simulink library "Diesel_Genset_lib"  (R2013a)
settings: Solver=ode45  StartTime=0.0  StopTime=10.0  RelTol=1e-3
undefined symbols (not defined in the file or in its folder): DiscIntNeverNeededParam, fdesignblkfcn, gcbh, ph, Ts
libraries: simulink x19, rtio_opalrt_common x19, powerlib x18, discretizing x4, rteventslib x4, simulink_extras x3, powerlib_extras x1, NG_Genset_lib x1
(part 1 of 3)
settings Model: Creator=ed12083  LastModifiedBy=ed12083

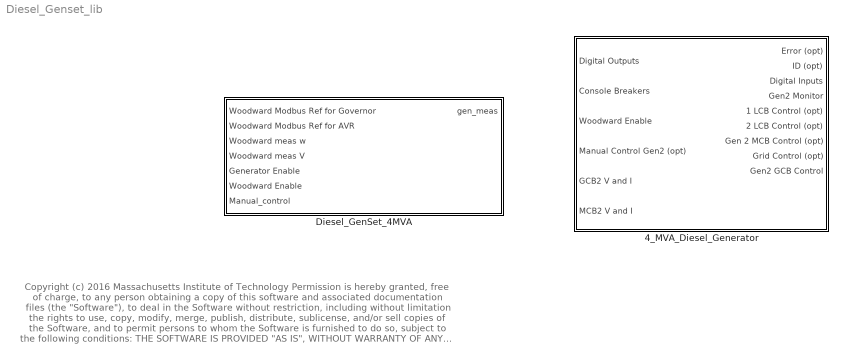
== system Diesel_Genset_lib ==
  note: Copyright (c) 2016 Massachusetts Institute of Technology
      | Permission is hereby granted, free of charge, to any person obtaining a copy of this software and associated documentation files (the "Software"), to deal
      | in the Software without restriction, including without limitation the rights to use, copy, modify, merge, publish, distribute, sublicense, and/or sell copies of the
      | Software, and to permit persons to whom the Software is furnished to do so, subject to the following conditions:
      |
      | THE SOFTWARE IS PROVIDED "AS IS", WITHOUT WARRANTY OF ANY KIND, EXPRESS OR IMPLIED, INCLUDING BUT NOT LIMITED TO THE
      | WARRANTIES OF MERCHANTABILITY, FITNESS FOR A PARTICULAR PURPOSE AND NONINFRINGEMENT. IN NO EVENT SHALL THE AUTHORS
      | OR COPYRIGHT HOLDERS BE LIABLE FOR ANY CLAIM, DAMAGES OR OTHER LIABILITY, WHETHER IN AN ACTION OF CONTRACT, TORT OR
      | OTHERWISE, ARISING FROM, OUT OF OR IN CONNECTION WITH THE SOFTWARE OR THE USE OR OTHER DEALINGS IN THE SOFTWARE.
  4_MVA_Diesel_Generator : Subsystem
  Diesel_GenSet_4MVA : Subsystem  mask(Gen-Set with simulated control modes){control_mode=1}
      mask prompts: control_mode "Control Mode [0 => Sim. 1 => Wood.]"
      mask help:
      | This Gen-Set block allows the user to indicate the control mode of the generator. The available control modes are: (1) PQ, (2) PV, and (3) VF.
      | The input values to the block will be applied according to the selected control mode.
      | For example, if PQ mode is selected, the controller will only work based on P_ref and Q_ref ignoring values of other inputs to the block.

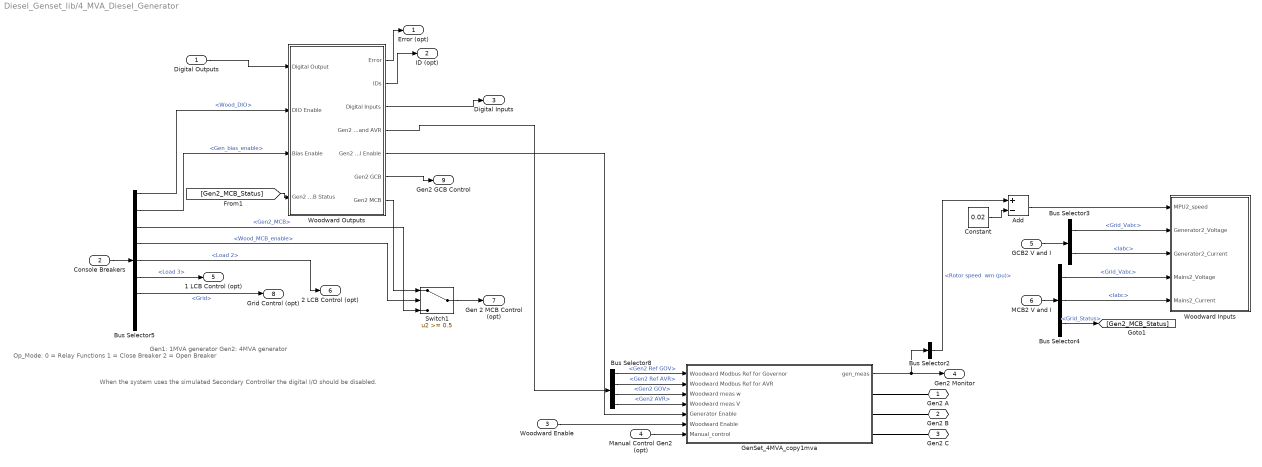
== system Diesel_Genset_lib/4_MVA_Diesel_Generator ==
  note: When the system uses the simulated
      | Secondary Controller the digital I/O
      | should be disabled.
  note: Gen1: 1MVA generator
      | Gen2: 4MVA generator
  note: Op_Mode:
      | 0 = Relay Functions
      | 1 = Close Breaker
      | 2 = Open Breaker
  Digital Outputs : Inport
  Console Breakers : Inport  Port=2
  Woodward Enable : Inport  Port=3
  Manual Control Gen2 (opt) : Inport  Port=4
  GCB2 V and I : Inport  Port=5
  MCB2 V and I : Inport  Port=6
  Add : Sum  Inputs=+-
  Bus Selector2 : BusSelector  OutputSignals="w.w.Rotor speed  wm (pu)"
  Bus Selector3 : BusSelector  OutputSignals=sel_787.Grid_Vabc,sel_787.Iabc
  Bus Selector4 : BusSelector  OutputSignals=sel_787.Grid_Vabc,sel_787.Iabc,Grid_Status
  Bus Selector5 : BusSelector  OutputSignals=Wood_DIO,Gen_bias_enable,Gen2_MCB,Wood_MCB_enable,Load 2,Load 3,Grid,Gen2_enable,Load 1
  Bus Selector8 : BusSelector  OutputSignals=Gen2 Ref GOV,Gen2 Ref AVR,Gen2 GOV,Gen2 AVR
  Constant : Constant  Value=0.02
  GenSet_4MVA_copy1mva : Subsystem  mask(Gen-Set with simulated control modes){control_mode=1}
      mask prompts: control_mode "Control Mode [0 => Sim. 1 => Wood.]"
      mask help:
      | This Gen-Set block allows the user to indicate the control mode of the generator. The available control modes are: (1) PQ, (2) PV, and (3) VF.
      | The input values to the block will be applied according to the selected control mode.
      | For example, if PQ mode is selected, the controller will only work based on P_ref and Q_ref ignoring values of other inputs to the block.
  Switch1 : Switch  Threshold=0.5
  Woodward Inputs : Subsystem
  Woodward Outputs : Subsystem
  Gen2 A : PMIOPort  Port=1  Side=Right
  Gen2 B : PMIOPort  Port=2  Side=Right
  Gen2 C : PMIOPort  Port=3  Side=Right
  Error (opt) : Outport
  ID (opt) : Outport  Port=2
  Digital Inputs : Outport  Port=3
  Gen2 Monitor : Outport  Port=4
  1 LCB Control (opt) : Outport  Port=5
  2 LCB Control (opt) : Outport  Port=6
  Gen 2 MCB Control (opt) : Outport  Port=7
  Grid Control (opt) : Outport  Port=8
  Gen2 GCB Control : Outport  Port=9
  wires:
  Bus Selector2/1 -> Add/1  "<Rotor speed  wm (pu)>"
  Bus Selector5/7 -> Grid Control (opt)/1  "<Grid>"
  Bus Selector5/3 -> Switch1/3  "<Gen2_MCB>"
  Bus Selector5/5 -> 2 LCB Control (opt)/1  "<Load 2>"
  Woodward Outputs/7(Gen2 MCB) -> Switch1/1
  Switch1/1 -> Gen 2 MCB Control (opt)/1
  [Gen2_MCB_Status] -> Woodward Outputs/4(Gen2 MCB Status)
  Bus Selector4/3 -> [Gen2_MCB_Status]  "<Grid_Status>"
  Constant/1 -> Add/2
  Add/1 -> Woodward Inputs/1(MPU2_speed)
  Woodward Outputs/6(Gen2 GCB) -> Gen2 GCB Control/1
  Woodward Outputs/5(Gen2 Fuel Enable) -> GenSet_4MVA_copy1mva/5(Generator Enable)
  Manual Control Gen2 (opt)/1 -> GenSet_4MVA_copy1mva/7(Manual_control)
  Bus Selector8/4 -> GenSet_4MVA_copy1mva/4(Woodward meas V)  "<Gen2 AVR>"
  Bus Selector8/3 -> GenSet_4MVA_copy1mva/3(Woodward meas w)  "<Gen2 GOV>"
  Bus Selector8/2 -> GenSet_4MVA_copy1mva/2(Woodward Modbus Ref for AVR)  "<Gen2 Ref AVR>"
  Bus Selector8/1 -> GenSet_4MVA_copy1mva/1(Woodward Modbus Ref for Governor)  "<Gen2 Ref GOV>"
  Woodward Outputs/4(Gen2 Gov and AVR) -> Bus Selector8/1
  Bus Selector4/2 -> Woodward Inputs/5(Mains2_Current)  "<Iabc>"
  Bus Selector4/1 -> Woodward Inputs/4(Mains2_Voltage)  "<Grid_Vabc>"
  Bus Selector3/2 -> Woodward Inputs/3(Generator2_Current)  "<Iabc>"
  Bus Selector3/1 -> Woodward Inputs/2(Generator2_Voltage)  "<Grid_Vabc>"
  GenSet_4MVA_copy1mva/1(gen_meas) -> Gen2 Monitor/1, Bus Selector2/1
  MCB2 V and I/1 -> Bus Selector4/1
  GCB2 V and I/1 -> Bus Selector3/1
  Bus Selector5/6 -> 1 LCB Control (opt)/1  "<Load 3>"
  Console Breakers/1 -> Bus Selector5/1
  Digital Outputs/1 -> Woodward Outputs/1(Digital Output)
  Bus Selector5/4 -> Switch1/2  "<Wood_MCB_enable>"
  Woodward Enable/1 -> GenSet_4MVA_copy1mva/6(Woodward Enable)
  Woodward Outputs/3(Digital Inputs) -> Digital Inputs/1
  Woodward Outputs/2(IDs) -> ID (opt)/1
  Woodward Outputs/1(Error) -> Error (opt)/1
  Bus Selector5/2 -> Woodward Outputs/3(Bias Enable)  "<Gen_bias_enable>"
  Bus Selector5/1 -> Woodward Outputs/2(DIO Enable)  "<Wood_DIO>"
  connections:
  Gen2 C/RConn1 -- GenSet_4MVA_copy1mva/RConn3
  GenSet_4MVA_copy1mva/RConn2 -- Gen2 B/RConn1
  Gen2 A/RConn1 -- GenSet_4MVA_copy1mva/RConn1

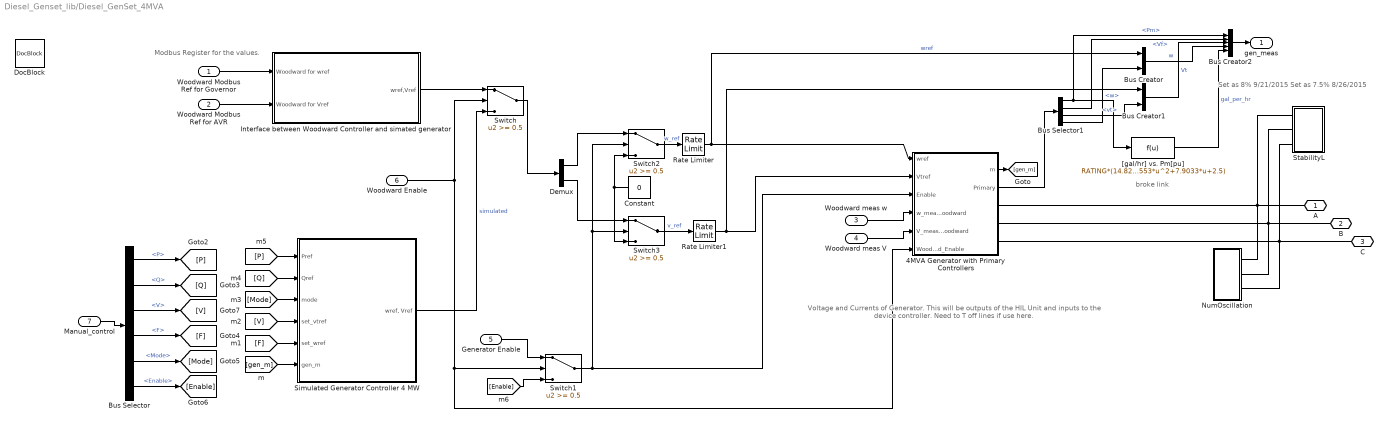
== system Diesel_Genset_lib/Diesel_GenSet_4MVA ==
  note: Modbus Register for the values.
  note: Voltage and Currents of Generator.
      | This will be outputs of the HIL Unit
      | and inputs to the device controller.
      | Need to T off lines if use here.
  note: Set as 8% 9/21/2015
      | Set as 7.5% 8/26/2015
  note: broke link
  Woodward Modbus Ref for Governor : Inport
  Woodward Modbus Ref for AVR : Inport  Port=2
  Woodward meas w : Inport  Port=3
  Woodward meas V : Inport  Port=4
  Generator Enable : Inport  Port=5
  Woodward Enable : Inport  Port=6
  Manual_control : Inport  Port=7
  4MVA Generator with Primary Controllers : Subsystem
  Bus Creator : BusCreator  Inputs=2
  Bus Creator1 : BusCreator  Inputs=2
  Bus Creator2 : BusCreator  Inputs=5
  Bus Selector : BusSelector  OutputSignals=P,Q,V,F,Mode,Enable
  Bus Selector1 : BusSelector  OutputSignals=Pm,Vf,vt,w
  Constant : Constant  Value=0
  Demux : Demux  Outputs=2
  DocBlock : simulink/Model-Wide Utilities/DocBlock  DocumentType=Text
      content=|
      | Author: Mirjana Marden, May 2015
      |
      | This is the model of 60kW generator with AVR and Governor.
      | There are two modes for controller implementation:
      |     1. Hardware implemented Woodward controller
      |     2. Simulated Generator Controller
      |
      | 1. Hardware implemented Woodward controller's output signals are DC voltages for both bias signals.
      |    The voltage range is -10 to 10V.
      |    The commanded reference values for generator frequency and voltage are wref and Vref.
      |    Interface between Woodward controller and simulation is a block that scales the bias signals.
      | 2. Simulated generator controller has three modes PQ, Vf and PV
  Interface between Woodward Controller and simated generator : Subsystem
  NumOscillation : Subsystem
  Rate Limiter : RateLimiter  RisingSlewLimit=0.5  FallingSlewLimit=-0.5  SampleTimeMode=inherited
  Rate Limiter1 : RateLimiter  RisingSlewLimit=0.5  FallingSlewLimit=-0.5  SampleTimeMode=inherited
  Simulated Generator Controller 4 MW : Subsystem
  StabilityL : Subsystem  mask{v=13800, kVA=320, pf=1}
  Switch{,1..3} (4 alike) : Switch  Threshold=0.5
  "[gal/hr] vs. Pm[pu]" : Fcn  Expr=RATING*(14.827*u^4-27.253*u^3+15.553*u^2+7.9033*u+2.5)  mask{RATING=4}
      mask prompts: RATING "Rating [MW]"
      mask help: This block computes the gal/hr vs Pm[pu] of a generator of a given rating [MW].
  A : PMIOPort  Port=1  Side=Right
  B : PMIOPort  Port=2  Side=Right
  C : PMIOPort  Port=3  Side=Right
  gen_meas : Outport
  wires:
  [F] -> Simulated Generator Controller 4 MW/5(set_wref)
  [V] -> Simulated Generator Controller 4 MW/4(set_vtref)
  [Mode] -> Simulated Generator Controller 4 MW/3(mode)
  [Q] -> Simulated Generator Controller 4 MW/2(Qref)
  [P] -> Simulated Generator Controller 4 MW/1(Pref)
  [gen_m] -> Simulated Generator Controller 4 MW/6(gen_m)
  Bus Selector/5 -> [Mode]  "<Mode>"
  Bus Selector/4 -> [F]  "<F>"
  Bus Selector/3 -> [V]  "<V>"
  Bus Selector/2 -> [Q]  "<Q>"
  Bus Selector/1 -> [P]  "<P>"
  Manual_control/1 -> Bus Selector/1
  Simulated Generator Controller 4 MW/1("wref, Vref") -> Switch/3  "simulated"
  4MVA Generator with Primary Controllers/1(m) -> [gen_m]
  Interface between Woodward Controller and simated generator/1(wref,Vref) -> Switch/1
  Switch/1 -> Demux/1
  Woodward Modbus Ref for Governor/1 -> Interface between Woodward Controller and simated generator/1(Woodward for wref)
  Woodward Modbus Ref for AVR/1 -> Interface between Woodward Controller and simated generator/2(Woodward for Vref)
  Woodward meas w/1 -> 4MVA Generator with Primary Controllers/4(w_meas_Woodward)
  Woodward meas V/1 -> 4MVA Generator with Primary Controllers/5(V_meas_Woodward)
  Bus Selector/6 -> [Enable]  "<Enable>"
  4MVA Generator with Primary Controllers/2(Primary) -> Bus Selector1/1
  Generator Enable/1 -> Switch1/1
  [Enable] -> Switch1/3
  Switch1/1 -> 4MVA Generator with Primary Controllers/3(Enable), Switch2/2, Switch3/2
  Switch2/1 -> Rate Limiter/1  "w_ref"
  Demux/1 -> Switch2/1
  Demux/2 -> Switch3/1
  Constant/1 -> Switch3/3, Switch2/3
  Switch3/1 -> Rate Limiter1/1  "v_ref"
  Bus Selector1/3 -> Bus Creator1/2  "<vt>"
  Bus Selector1/4 -> Bus Creator/2  "<w>"
  Bus Selector1/2 -> Bus Creator2/2  "<Vf>"
  Bus Selector1/1 -> Bus Creator2/1, "[gal/hr] vs. Pm[pu]"/1  "<Pm>"
  Bus Creator1/1 -> Bus Creator2/3  "Vt"
  Bus Creator/1 -> Bus Creator2/4  "w"
  Bus Creator2/1 -> gen_meas/1
  Rate Limiter/1 -> 4MVA Generator with Primary Controllers/1(wref), Bus Creator/1  "wref"
  Rate Limiter1/1 -> 4MVA Generator with Primary Controllers/2(Vtref), Bus Creator1/1
  Woodward Enable/1 -> Switch/2, Switch1/2, 4MVA Generator with Primary Controllers/6(Woodward_Enable)
  "[gal/hr] vs. Pm[pu]"/1 -> Bus Creator2/5  "gal_per_hr"
  connections:
  StabilityL/LConn1 -- A/RConn1 -- 4MVA Generator with Primary Controllers/RConn1 -- NumOscillation/LConn1
  StabilityL/LConn2 -- 4MVA Generator with Primary Controllers/RConn2 -- B/RConn1 -- NumOscillation/LConn2
  StabilityL/LConn3 -- C/RConn1 -- 4MVA Generator with Primary Controllers/RConn3 -- NumOscillation/LConn3

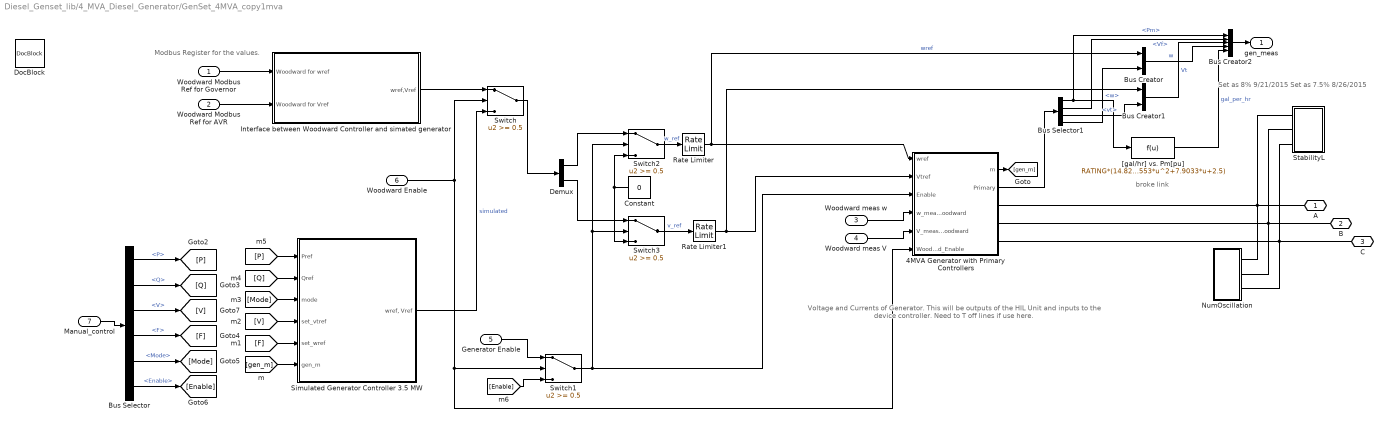
== system Diesel_Genset_lib/4_MVA_Diesel_Generator/GenSet_4MVA_copy1mva ==
  note: Modbus Register for the values.
  note: Voltage and Currents of Generator.
      | This will be outputs of the HIL Unit
      | and inputs to the device controller.
      | Need to T off lines if use here.
  note: Set as 8% 9/21/2015
      | Set as 7.5% 8/26/2015
  note: broke link
  Woodward Modbus Ref for Governor : Inport
  Woodward Modbus Ref for AVR : Inport  Port=2
  Woodward meas w : Inport  Port=3
  Woodward meas V : Inport  Port=4
  Generator Enable : Inport  Port=5
  Woodward Enable : Inport  Port=6
  Manual_control : Inport  Port=7
  4MVA Generator with Primary Controllers : Subsystem
  Bus Creator : BusCreator  Inputs=2
  Bus Creator1 : BusCreator  Inputs=2
  Bus Creator2 : BusCreator  Inputs=5
  Bus Selector : BusSelector  OutputSignals=P,Q,V,F,Mode,Enable
  Bus Selector1 : BusSelector  OutputSignals=Pm,Vf,vt,w
  Constant : Constant  Value=0
  Demux : Demux  Outputs=2
  DocBlock : simulink/Model-Wide Utilities/DocBlock  DocumentType=Text
      content=|
      | Author: Mirjana Marden, May 2015
      |
      | This is the model of 60kW generator with AVR and Governor.
      | There are two modes for controller implementation:
      |     1. Hardware implemented Woodward controller
      |     2. Simulated Generator Controller
      |
      | 1. Hardware implemented Woodward controller's output signals are DC voltages for both bias signals.
      |    The voltage range is -10 to 10V.
      |    The commanded reference values for generator frequency and voltage are wref and Vref.
      |    Interface between Woodward controller and simulation is a block that scales the bias signals.
      | 2. Simulated generator controller has three modes PQ, Vf and PV
  Interface between Woodward Controller and simated generator : Subsystem
  NumOscillation : Subsystem
  Rate Limiter : RateLimiter  RisingSlewLimit=0.5  FallingSlewLimit=-0.5  SampleTimeMode=inherited
  Rate Limiter1 : RateLimiter  RisingSlewLimit=0.5  FallingSlewLimit=-0.5  SampleTimeMode=inherited
  Simulated Generator Controller 3.5 MW : Subsystem
  StabilityL : Subsystem  mask{v=13800, kVA=320, pf=1}
  Switch{,1..3} (4 alike) : Switch  Threshold=0.5
  "[gal/hr] vs. Pm[pu]" : Fcn  Expr=RATING*(14.827*u^4-27.253*u^3+15.553*u^2+7.9033*u+2.5)  mask{RATING=4}
      mask prompts: RATING "Rating [MW]"
      mask help: This block computes the gal/hr vs Pm[pu] of a generator of a given rating [MW].
  A : PMIOPort  Port=1  Side=Right
  B : PMIOPort  Port=2  Side=Right
  C : PMIOPort  Port=3  Side=Right
  gen_meas : Outport
  wires:
  [F] -> Simulated Generator Controller 3.5 MW/5(set_wref)
  [V] -> Simulated Generator Controller 3.5 MW/4(set_vtref)
  [Mode] -> Simulated Generator Controller 3.5 MW/3(mode)
  [Q] -> Simulated Generator Controller 3.5 MW/2(Qref)
  [P] -> Simulated Generator Controller 3.5 MW/1(Pref)
  [gen_m] -> Simulated Generator Controller 3.5 MW/6(gen_m)
  Bus Selector/5 -> [Mode]  "<Mode>"
  Bus Selector/4 -> [F]  "<F>"
  Bus Selector/3 -> [V]  "<V>"
  Bus Selector/2 -> [Q]  "<Q>"
  Bus Selector/1 -> [P]  "<P>"
  Manual_control/1 -> Bus Selector/1
  Simulated Generator Controller 3.5 MW/1("wref, Vref") -> Switch/3  "simulated"
  4MVA Generator with Primary Controllers/1(m) -> [gen_m]
  Interface between Woodward Controller and simated generator/1(wref,Vref) -> Switch/1
  Switch/1 -> Demux/1
  Woodward Modbus Ref for Governor/1 -> Interface between Woodward Controller and simated generator/1(Woodward for wref)
  Woodward Modbus Ref for AVR/1 -> Interface between Woodward Controller and simated generator/2(Woodward for Vref)
  Woodward meas w/1 -> 4MVA Generator with Primary Controllers/4(w_meas_Woodward)
  Woodward meas V/1 -> 4MVA Generator with Primary Controllers/5(V_meas_Woodward)
  Bus Selector/6 -> [Enable]  "<Enable>"
  4MVA Generator with Primary Controllers/2(Primary) -> Bus Selector1/1
  Generator Enable/1 -> Switch1/1
  [Enable] -> Switch1/3
  Switch1/1 -> 4MVA Generator with Primary Controllers/3(Enable), Switch2/2, Switch3/2
  Switch2/1 -> Rate Limiter/1  "w_ref"
  Demux/1 -> Switch2/1
  Demux/2 -> Switch3/1
  Constant/1 -> Switch3/3, Switch2/3
  Switch3/1 -> Rate Limiter1/1  "v_ref"
  Bus Selector1/3 -> Bus Creator1/2  "<vt>"
  Bus Selector1/4 -> Bus Creator/2  "<w>"
  Bus Selector1/2 -> Bus Creator2/2  "<Vf>"
  Bus Selector1/1 -> Bus Creator2/1, "[gal/hr] vs. Pm[pu]"/1  "<Pm>"
  Bus Creator1/1 -> Bus Creator2/3  "Vt"
  Bus Creator/1 -> Bus Creator2/4  "w"
  Bus Creator2/1 -> gen_meas/1
  Rate Limiter/1 -> 4MVA Generator with Primary Controllers/1(wref), Bus Creator/1  "wref"
  Rate Limiter1/1 -> 4MVA Generator with Primary Controllers/2(Vtref), Bus Creator1/1
  Woodward Enable/1 -> Switch/2, Switch1/2, 4MVA Generator with Primary Controllers/6(Woodward_Enable)
  "[gal/hr] vs. Pm[pu]"/1 -> Bus Creator2/5  "gal_per_hr"
  connections:
  StabilityL/LConn1 -- A/RConn1 -- 4MVA Generator with Primary Controllers/RConn1 -- NumOscillation/LConn1
  StabilityL/LConn2 -- 4MVA Generator with Primary Controllers/RConn2 -- B/RConn1 -- NumOscillation/LConn2
  StabilityL/LConn3 -- C/RConn1 -- 4MVA Generator with Primary Controllers/RConn3 -- NumOscillation/LConn3

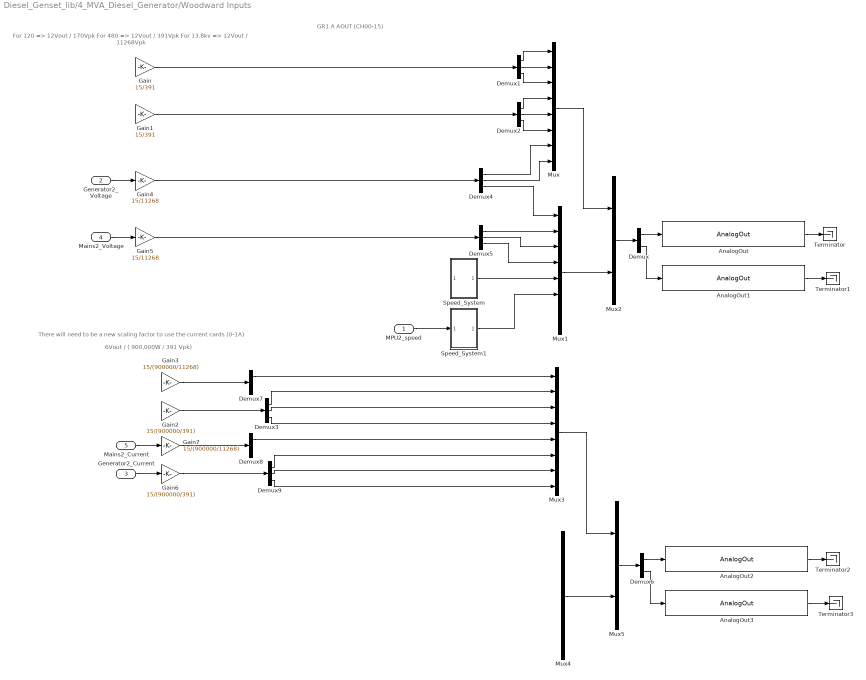
== system Diesel_Genset_lib/4_MVA_Diesel_Generator/Woodward Inputs ==
  note: There will need to be a
      | new scaling factor to use
      | the current cards (0-1A)
  note: GR1 A AOUT (CH00-15)
  note: For 120 => 12Vout / 170Vpk
      | For 480 => 12Vout / 391Vpk
      | For 13.8kv => 12Vout / 11268Vpk
  note: 6Vout / ( 900,000W / 391 Vpk)
  MPU2_speed : Inport
  Generator2_Voltage : Inport  Port=2
  Generator2_Current : Inport  Port=3
  Mains2_Voltage : Inport  Port=4
  Mains2_Current : Inport  Port=5
  AnalogOut : rtio_opalrt_common/AnalogOut  CtrlName='OpCtrl'  portNb=1  FcnNos=Slot 1 Module A Subsection 1  size=16  maxcount=8  count=8  numchan=8  israngeinput=off  voltagerange=[-16 ... 16]  slot=0  side=0  mismatch=0  slotside=Slot_1_Module_A
      settings: AttributesFormatString=%<CtrlName>
  AnalogOut1 : rtio_opalrt_common/AnalogOut  CtrlName='OpCtrl'  portNb=2  FcnNos=Slot 1 Module A Subsection 2  size=16  maxcount=8  count=8  numchan=8  israngeinput=off  voltagerange=[-16 ... 16]  slot=0  side=0  mismatch=0  slotside=Slot_1_Module_A
      settings: AttributesFormatString=%<CtrlName>
  AnalogOut2 : rtio_opalrt_common/AnalogOut  CtrlName='OpCtrl'  portNb=3  FcnNos=Slot 2 Module A Subsection 1  size=16  maxcount=8  count=8  numchan=8  israngeinput=off  voltagerange=[-16 ... 16]  slot=1  side=0  mismatch=0  slotside=Slot_2_Module_A
      settings: AttributesFormatString=%<CtrlName>
  AnalogOut3 : rtio_opalrt_common/AnalogOut  CtrlName='OpCtrl'  portNb=4  FcnNos=Slot 2 Module A Subsection 2  size=16  maxcount=8  count=8  numchan=8  israngeinput=off  voltagerange=[-16 ... 16]  slot=1  side=0  mismatch=0  slotside=Slot_2_Module_A
      settings: AttributesFormatString=%<CtrlName>
  Demux : Demux  Outputs=2
  Demux{1..5,7..9} (8 alike) : Demux  Outputs=3
  Demux6 : Demux  Outputs=2
  Gain : Gain  Gain=15/391
  Gain1 : Gain  Gain=15/391
  Gain2 : Gain  Gain=15/(900000/391)
  Gain3 : Gain  Gain=15/(900000/11268)
  Gain4 : Gain  Gain=15/11268
  Gain5 : Gain  Gain=15/11268
  Gain6 : Gain  Gain=15/(900000/391)
  Gain7 : Gain  Gain=15/(900000/11268)
  Mux{,1,3..4} (4 alike) : Mux  Inputs=8
  Mux2 : Mux  Inputs=2
  Mux5 : Mux  Inputs=2
  Speed_System : Subsystem
  Speed_System1 : Subsystem
  Terminator{,1..3} (4 alike) : Terminator
  wires:
  Demux9/3 -> Mux3/8
  Demux9/2 -> Mux3/7
  Demux9/1 -> Mux3/6
  Gain6/1 -> Demux9/1
  Demux8/1 -> Mux3/5
  Gain7/1 -> Demux8/1
  Mains2_Current/1 -> Gain7/1
  Generator2_Current/1 -> Gain6/1
  Speed_System1/1(Out1) -> Mux1/6
  MPU2_speed/1 -> Speed_System1/1(In1)
  Generator2_Voltage/1 -> Gain4/1
  Mains2_Voltage/1 -> Gain5/1
  Gain4/1 -> Demux4/1
  Gain5/1 -> Demux5/1
  Demux7/1 -> Mux3/1
  Gain3/1 -> Demux7/1
  ? -> Gain3/1
  Demux3/3 -> Mux3/4
  Demux3/2 -> Mux3/3
  Demux3/1 -> Mux3/2
  Gain2/1 -> Demux3/1
  AnalogOut2/1 -> Terminator2/1
  AnalogOut3/1 -> Terminator3/1
  Demux6/1 -> AnalogOut2/1
  Demux6/2 -> AnalogOut3/1
  Mux3/1 -> Mux5/1
  Mux4/1 -> Mux5/2
  Mux5/1 -> Demux6/1
  Demux5/3 -> Mux1/4
  Demux5/2 -> Mux1/3
  Demux5/1 -> Mux1/2
  Demux4/3 -> Mux1/1
  Demux4/2 -> Mux/8
  Demux4/1 -> Mux/7
  Speed_System/1(Out1) -> Mux1/5
  Demux2/3 -> Mux/6
  Demux2/2 -> Mux/5
  Demux2/1 -> Mux/4
  Demux1/3 -> Mux/3
  Demux1/2 -> Mux/2
  Demux1/1 -> Mux/1
  AnalogOut/1 -> Terminator/1
  AnalogOut1/1 -> Terminator1/1
  Demux/1 -> AnalogOut/1
  Demux/2 -> AnalogOut1/1
  ? -> Gain/1
  Mux/1 -> Mux2/1
  Mux1/1 -> Mux2/2
  Mux2/1 -> Demux/1
  ? -> Gain1/1
  Gain/1 -> Demux1/1
  Gain1/1 -> Demux2/1
  ? -> Gain2/1
  ? -> Speed_System/1(In1)

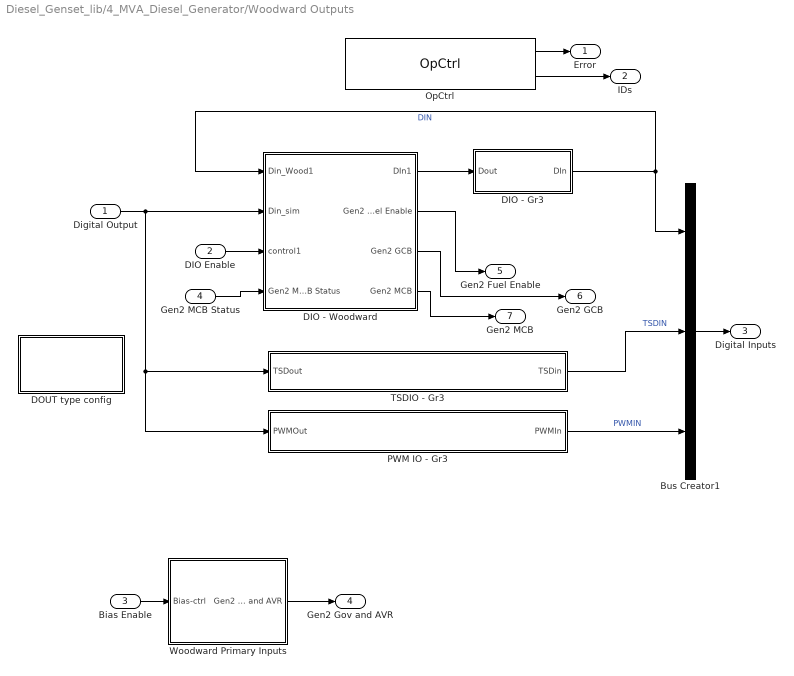
== system Diesel_Genset_lib/4_MVA_Diesel_Generator/Woodward Outputs ==
  Digital Output : Inport
  DIO Enable : Inport  Port=2
  Bias Enable : Inport  Port=3
  Gen2 MCB Status : Inport  Port=4
  Bus Creator1 : BusCreator  Inputs=3
  DIO - Gr3 : Subsystem
  DIO - Woodward : Subsystem
  DOUT type config : Subsystem
  OpCtrl : rtio_opalrt_common/OpCtrl  CtrlName='OpCtrl'  boardid=0  BitstreamFilename=VC707_2-EX-0001-2_2_6_61-32AIO16DIO16DIOSel-01-01.bin  numconfig=-1  mode=Master  externalClock=off  decimRtsi=0  calibIO=off  SampleTime=0  loadinport=-1  BoardType=VC707  SecondaryPresent=off  sync_type=Audio
  PWM IO - Gr3 : Subsystem
  TSDIO - Gr3 : Subsystem
  Woodward Primary Inputs : Subsystem
  Error : Outport
  IDs : Outport  Port=2
  Digital Inputs : Outport  Port=3
  Gen2 Gov and AVR : Outport  Port=4
  Gen2 Fuel Enable : Outport  Port=5
  Gen2 GCB : Outport  Port=6
  Gen2 MCB : Outport  Port=7
  wires:
  Gen2 MCB Status/1 -> DIO - Woodward/4(Gen2 MCB Status)
  DIO - Woodward/4(Gen2 MCB) -> Gen2 MCB/1
  DIO - Woodward/2(Gen2 Fuel Enable) -> Gen2 Fuel Enable/1
  DIO - Woodward/3(Gen2 GCB) -> Gen2 GCB/1
  Digital Output/1 -> TSDIO - Gr3/1(TSDout), PWM IO - Gr3/1(PWMOut), DIO - Woodward/2(Din_sim)
  Bias Enable/1 -> Woodward Primary Inputs/1(Bias-ctrl)
  Woodward Primary Inputs/1(Gen2 Gov and AVR) -> Gen2 Gov and AVR/1
  DIO Enable/1 -> DIO - Woodward/3(control1)
  Bus Creator1/1 -> Digital Inputs/1
  DIO - Gr3/1(DIn) -> DIO - Woodward/1(Din_Wood1), Bus Creator1/1  "DIN"
  TSDIO - Gr3/1(TSDin) -> Bus Creator1/2  "TSDIN"
  PWM IO - Gr3/1(PWMIn) -> Bus Creator1/3  "PWMIN"
  DIO - Woodward/1(DIn1) -> DIO - Gr3/1(Dout)
  OpCtrl/2 -> IDs/1
  OpCtrl/1 -> Error/1

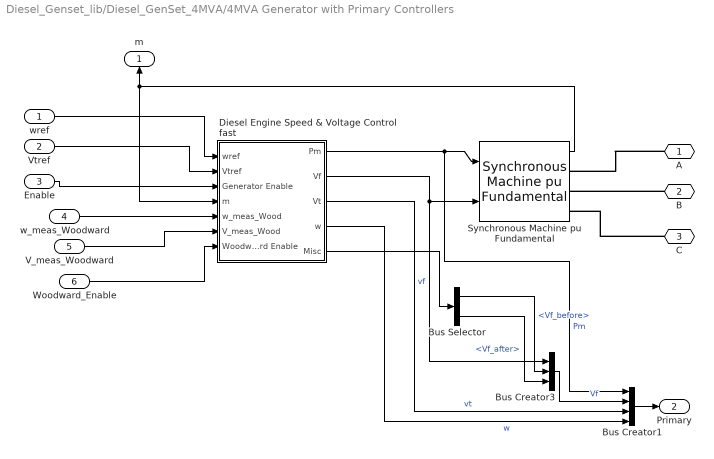
== system Diesel_Genset_lib/Diesel_GenSet_4MVA/4MVA Generator with Primary Controllers ==
  wref : Inport
  Vtref : Inport  Port=2
  Enable : Inport  Port=3
  w_meas_Woodward : Inport  Port=4
  V_meas_Woodward : Inport  Port=5
  Woodward_Enable : Inport  Port=6
  Bus Creator1 : BusCreator
  Bus Creator3 : BusCreator  Inputs=3
  Bus Selector : BusSelector  OutputSignals=Vf_before,Vf_after
  Diesel Engine Speed & Voltage Control fast : Subsystem
  Synchronous Machine pu Fundamental : powerlib/Machines/Synchronous Machine pu Fundamental  PresetModel=No  MechanicalLoad=Mechanical power Pm  ShowDetailedParameters=on  RotorType=Salient-pole  NominalParameters=[4e+006 13800 60]  Stator=[0.008979 0.05 2.35 1.72]  Field=[0.00206 0.511]  Dampers2=[0.0652, 0.5134, 0.0287, 0.2553, 7.765e-3, 0.9167 ]  Dampers1=[0.2826 3.738 0.02545 0.2392]  Mechanical=[0.3468 0.009238 2]  PolePairs=2  InitialConditions="[ -99  0  0  0  0  0  0  0  0 ]"  SetSaturation=off  Saturation=[0.6404,0.7127,0.8441,0.9214,0.9956,1.082,1.19,1.316,1.457;0.7,0.7698,0.8872,0.9466,0.9969,1.046,1.1,1.151,1.201]  Units=per unit fundamental parameters  LoadFlowParameters=[1,0,0,0,0]  TsPowergui=0  TsBlock=-1  IterativeModel=Forward Euler  BusType=swing  Pref=0  Qref=0  Qmin=-inf  Qmax=inf  PLF=0  QLF=0
  A : PMIOPort  Port=1  Side=Right
  B : PMIOPort  Port=2  Side=Right
  C : PMIOPort  Port=3  Side=Right
  m : Outport
  Primary : Outport  Port=2
  wires:
  Vtref/1 -> Diesel Engine Speed & Voltage Control fast/2(Vtref)
  wref/1 -> Diesel Engine Speed & Voltage Control fast/1(wref)
  Diesel Engine Speed & Voltage Control fast/2(Vf) -> Synchronous Machine pu Fundamental/2, Bus Creator3/1  "vf"
  Diesel Engine Speed & Voltage Control fast/1(Pm) -> Synchronous Machine pu Fundamental/1, Bus Creator1/1  "Pm"
  Enable/1 -> Diesel Engine Speed & Voltage Control fast/3(Generator Enable)
  Synchronous Machine pu Fundamental/1 -> m/1, Diesel Engine Speed & Voltage Control fast/4(m)
  w_meas_Woodward/1 -> Diesel Engine Speed & Voltage Control fast/5(w_meas_Wood)
  V_meas_Woodward/1 -> Diesel Engine Speed & Voltage Control fast/6(V_meas_Wood)
  Diesel Engine Speed & Voltage Control fast/3(Vt) -> Bus Creator1/3  "vt"
  Diesel Engine Speed & Voltage Control fast/4(w) -> Bus Creator1/4  "w"
  Bus Creator1/1 -> Primary/1
  Diesel Engine Speed & Voltage Control fast/5(Misc) -> Bus Selector/1
  Bus Selector/1 -> Bus Creator3/2  "<Vf_before>"
  Bus Selector/2 -> Bus Creator3/3  "<Vf_after>"
  Bus Creator3/1 -> Bus Creator1/2  "Vf"
  Woodward_Enable/1 -> Diesel Engine Speed & Voltage Control fast/7(Woodward Enable)
  connections:
  C/RConn1 -- Synchronous Machine pu Fundamental/RConn3
  B/RConn1 -- Synchronous Machine pu Fundamental/RConn2
  A/RConn1 -- Synchronous Machine pu Fundamental/RConn1

== system Diesel_Genset_lib/Diesel_GenSet_4MVA/Interface between Woodward Controller and simated generator ==
  note: Note: This may need a different scaling because it is the reference signal.
      | Reference has to be between 0.95 and 1.05 pu in order to be in tolerance.
  Woodward for wref : Inport
  Woodward for Vref : Inport  Port=2
  Add2 : Sum
  Add3 : Sum
  Gain2 : Gain
  Gain3 : Gain
  Mux1 : Mux  Inputs=2
  Vref_set : Constant  Value=0
  wref_set : Constant  Value=0
  wref,Vref : Outport
  wires:
  Gain2/1 -> Add2/1  "bias"
  Add2/1 -> Mux1/1
  wref_set/1 -> Add2/2
  Gain3/1 -> Add3/1  "bias"
  Vref_set/1 -> Add3/2
  Add3/1 -> Mux1/2
  Woodward for wref/1 -> Gain2/1
  Mux1/1 -> wref,Vref/1  "hardware"
  Woodward for Vref/1 -> Gain3/1

== system Diesel_Genset_lib/Diesel_GenSet_4MVA/NumOscillation ==
  Ground2 : powerlib/Elements/Ground  LConnTagsString=a
  "RLC " : powerlib/Elements/Parallel RLC Branch  LConnTagsString=a  RConnTagsString=__new0  BranchType=R  Resistance=10e6  Inductance=inf  SetiL0=off  InitialCurrent=0  Capacitance=10e-6  Setx0=off  InitialVoltage=0  Measurements=None
  RLC1 : powerlib/Elements/Parallel RLC Branch  LConnTagsString=a  RConnTagsString=__new0  BranchType=R  Resistance=10e6  Inductance=inf  SetiL0=off  InitialCurrent=0  Capacitance=10e-6  Setx0=off  InitialVoltage=0  Measurements=None
  RLC2 : powerlib/Elements/Parallel RLC Branch  LConnTagsString=a  RConnTagsString=__new0  BranchType=R  Resistance=10e6  Inductance=inf  SetiL0=off  InitialCurrent=0  Capacitance=10e-6  Setx0=off  InitialVoltage=0  Measurements=None
  RLC3 : powerlib/Elements/Parallel RLC Branch  LConnTagsString=a  RConnTagsString=__new0  BranchType=R  Resistance=10e-3  Inductance=inf  SetiL0=off  InitialCurrent=0  Capacitance=0  Setx0=off  InitialVoltage=0  Measurements=None
  RLC4 : powerlib/Elements/Parallel RLC Branch  LConnTagsString=a  RConnTagsString=__new0  BranchType=R  Resistance=10e-3  Inductance=inf  SetiL0=off  InitialCurrent=0  Capacitance=0  Setx0=off  InitialVoltage=0  Measurements=None
  RLC5 : powerlib/Elements/Parallel RLC Branch  LConnTagsString=a  RConnTagsString=__new0  BranchType=R  Resistance=10e-3  Inductance=inf  SetiL0=off  InitialCurrent=0  Capacitance=0  Setx0=off  InitialVoltage=0  Measurements=None
  A : PMIOPort  Port=1  Side=Left
  B : PMIOPort  Port=2  Side=Left
  C : PMIOPort  Port=3  Side=Left
  connections:
  C/RConn1 -- RLC5/LConn1
  B/RConn1 -- RLC4/LConn1
  A/RConn1 -- RLC3/LConn1
  RLC3/RConn1 -- RLC2/LConn1
  RLC1/LConn1 -- RLC4/RConn1
  "RLC "/LConn1 -- RLC5/RConn1
  RLC2/RConn1 -- Ground2/LConn1 -- RLC1/RConn1 -- "RLC "/RConn1

== system Diesel_Genset_lib/Diesel_GenSet_4MVA/Simulated Generator Controller 4 MW ==
  Pref : Inport
  Qref : Inport  Port=2
  mode : Inport  Port=3
  set_vtref : Inport  Port=4
  set_wref : Inport  Port=5
  gen_m : Inport  Port=6
  Bus Selector1 : BusSelector  OutputSignals="Output active power   Peo (pu),Output reactive power  Qeo (pu)"
  Multiport Switch : MultiPortSwitch  DiagnosticForDefault=Warning
  Mux1 : Mux  Inputs=2
  Mux2 : Mux  Inputs=2
  Mux3 : Mux  Inputs=2
  PQ control : Subsystem
  PV control : Subsystem
  "wref, Vref" : Outport
  wires:
  Bus Selector1/1 -> PQ control/2(P (pu)), PV control/2(P (pu))  "<Output active power   Peo (pu)>"
  gen_m/1 -> Bus Selector1/1
  PQ control/1(w_ref (pu)) -> Mux1/1
  PQ control/2(V_ref (pu)) -> Mux1/2
  PV control/1(w_ref (pu)) -> Mux2/1
  set_vtref/1 -> Mux2/2, Mux3/2
  Mux1/1 -> Multiport Switch/2
  Mux2/1 -> Multiport Switch/3
  Mux3/1 -> Multiport Switch/4
  Pref/1 -> PQ control/1(P_ref (pu)), PV control/1(P_ref (pu))
  Bus Selector1/2 -> PQ control/4(Q (pu))  "<Output reactive power  Qeo (pu)>"
  set_wref/1 -> Mux3/1
  Qref/1 -> PQ control/3(Q_ref (pu))
  mode/1 -> Multiport Switch/1
  Multiport Switch/1 -> "wref, Vref"/1

== system Diesel_Genset_lib/Diesel_GenSet_4MVA/StabilityL ==
  Constant Load : powerlib/Elements/Three-Phase Parallel RLC Load  LConnTagsString=A|B|C  Configuration=Y (grounded)  NominalVoltage=v  NominalFrequency=60  ActivePower=kVA*1E3*pf  InductivePower=kVA*1E3*sqrt(1-pf^2)  CapacitivePower=0  Measurements=None  LoadType=constant Z
  A : PMIOPort  Port=1  Side=Left
  B : PMIOPort  Port=2  Side=Left
  C : PMIOPort  Port=3  Side=Left
  connections:
  A/RConn1 -- Constant Load/LConn1
  B/RConn1 -- Constant Load/LConn2
  C/RConn1 -- Constant Load/LConn3

== system Diesel_Genset_lib/4_MVA_Diesel_Generator/GenSet_4MVA_copy1mva/4MVA Generator with Primary Controllers ==
  wref : Inport
  Vtref : Inport  Port=2
  Enable : Inport  Port=3
  w_meas_Woodward : Inport  Port=4
  V_meas_Woodward : Inport  Port=5
  Woodward_Enable : Inport  Port=6
  Bus Creator1 : BusCreator
  Bus Creator3 : BusCreator  Inputs=3
  Bus Selector : BusSelector  OutputSignals=Vf_before,Vf_after
  Diesel Engine Speed & Voltage Control fast : Subsystem
  Synchronous Machine pu Fundamental : powerlib/Machines/Synchronous Machine pu Fundamental  PresetModel=No  MechanicalLoad=Mechanical power Pm  ShowDetailedParameters=on  RotorType=Salient-pole  NominalParameters=[4e+006 13800 60]  Stator=[0.008979 0.05 2.35 1.72]  Field=[0.00206 0.511]  Dampers2=[0.0652, 0.5134, 0.0287, 0.2553, 7.765e-3, 0.9167 ]  Dampers1=[0.2826 3.738 0.02545 0.2392]  Mechanical=[0.3468 0.009238 2]  PolePairs=2  InitialConditions="[ -99  0  0  0  0  0  0  0  0 ]"  SetSaturation=off  Saturation=[0.6404,0.7127,0.8441,0.9214,0.9956,1.082,1.19,1.316,1.457;0.7,0.7698,0.8872,0.9466,0.9969,1.046,1.1,1.151,1.201]  Units=per unit fundamental parameters  LoadFlowParameters=[1,0,0,0,0]  TsPowergui=0  TsBlock=-1  IterativeModel=Forward Euler  BusType=swing  Pref=0  Qref=0  Qmin=-inf  Qmax=inf  PLF=0  QLF=0
  A : PMIOPort  Port=1  Side=Right
  B : PMIOPort  Port=2  Side=Right
  C : PMIOPort  Port=3  Side=Right
  m : Outport
  Primary : Outport  Port=2
  wires:
  Vtref/1 -> Diesel Engine Speed & Voltage Control fast/2(Vtref)
  wref/1 -> Diesel Engine Speed & Voltage Control fast/1(wref)
  Diesel Engine Speed & Voltage Control fast/2(Vf) -> Synchronous Machine pu Fundamental/2, Bus Creator3/1  "vf"
  Diesel Engine Speed & Voltage Control fast/1(Pm) -> Synchronous Machine pu Fundamental/1, Bus Creator1/1  "Pm"
  Enable/1 -> Diesel Engine Speed & Voltage Control fast/3(Generator Enable)
  Synchronous Machine pu Fundamental/1 -> m/1, Diesel Engine Speed & Voltage Control fast/4(m)
  w_meas_Woodward/1 -> Diesel Engine Speed & Voltage Control fast/5(w_meas_Wood)
  V_meas_Woodward/1 -> Diesel Engine Speed & Voltage Control fast/6(V_meas_Wood)
  Diesel Engine Speed & Voltage Control fast/3(Vt) -> Bus Creator1/3  "vt"
  Diesel Engine Speed & Voltage Control fast/4(w) -> Bus Creator1/4  "w"
  Bus Creator1/1 -> Primary/1
  Diesel Engine Speed & Voltage Control fast/5(Misc) -> Bus Selector/1
  Bus Selector/1 -> Bus Creator3/2  "<Vf_before>"
  Bus Selector/2 -> Bus Creator3/3  "<Vf_after>"
  Bus Creator3/1 -> Bus Creator1/2  "Vf"
  Woodward_Enable/1 -> Diesel Engine Speed & Voltage Control fast/7(Woodward Enable)
  connections:
  C/RConn1 -- Synchronous Machine pu Fundamental/RConn3
  B/RConn1 -- Synchronous Machine pu Fundamental/RConn2
  A/RConn1 -- Synchronous Machine pu Fundamental/RConn1

== system Diesel_Genset_lib/4_MVA_Diesel_Generator/GenSet_4MVA_copy1mva/Interface between Woodward Controller and simated generator ==
  note: Note: This may need a different scaling because it is the reference signal.
      | Reference has to be between 0.95 and 1.05 pu in order to be in tolerance.
  Woodward for wref : Inport
  Woodward for Vref : Inport  Port=2
  Add2 : Sum
  Add3 : Sum
  Gain2 : Gain
  Gain3 : Gain
  Mux1 : Mux  Inputs=2
  Vref_set : Constant  Value=0
  wref_set : Constant  Value=0
  wref,Vref : Outport
  wires:
  Gain2/1 -> Add2/1  "bias"
  Add2/1 -> Mux1/1
  wref_set/1 -> Add2/2
  Gain3/1 -> Add3/1  "bias"
  Vref_set/1 -> Add3/2
  Add3/1 -> Mux1/2
  Woodward for wref/1 -> Gain2/1
  Mux1/1 -> wref,Vref/1  "hardware"
  Woodward for Vref/1 -> Gain3/1

== system Diesel_Genset_lib/4_MVA_Diesel_Generator/GenSet_4MVA_copy1mva/NumOscillation ==
  Ground2 : powerlib/Elements/Ground  LConnTagsString=a
  "RLC " : powerlib/Elements/Parallel RLC Branch  LConnTagsString=a  RConnTagsString=__new0  BranchType=R  Resistance=10e6  Inductance=inf  SetiL0=off  InitialCurrent=0  Capacitance=10e-6  Setx0=off  InitialVoltage=0  Measurements=None
  RLC1 : powerlib/Elements/Parallel RLC Branch  LConnTagsString=a  RConnTagsString=__new0  BranchType=R  Resistance=10e6  Inductance=inf  SetiL0=off  InitialCurrent=0  Capacitance=10e-6  Setx0=off  InitialVoltage=0  Measurements=None
  RLC2 : powerlib/Elements/Parallel RLC Branch  LConnTagsString=a  RConnTagsString=__new0  BranchType=R  Resistance=10e6  Inductance=inf  SetiL0=off  InitialCurrent=0  Capacitance=10e-6  Setx0=off  InitialVoltage=0  Measurements=None
  RLC3 : powerlib/Elements/Parallel RLC Branch  LConnTagsString=a  RConnTagsString=__new0  BranchType=R  Resistance=10e-3  Inductance=inf  SetiL0=off  InitialCurrent=0  Capacitance=0  Setx0=off  InitialVoltage=0  Measurements=None
  RLC4 : powerlib/Elements/Parallel RLC Branch  LConnTagsString=a  RConnTagsString=__new0  BranchType=R  Resistance=10e-3  Inductance=inf  SetiL0=off  InitialCurrent=0  Capacitance=0  Setx0=off  InitialVoltage=0  Measurements=None
  RLC5 : powerlib/Elements/Parallel RLC Branch  LConnTagsString=a  RConnTagsString=__new0  BranchType=R  Resistance=10e-3  Inductance=inf  SetiL0=off  InitialCurrent=0  Capacitance=0  Setx0=off  InitialVoltage=0  Measurements=None
  A : PMIOPort  Port=1  Side=Left
  B : PMIOPort  Port=2  Side=Left
  C : PMIOPort  Port=3  Side=Left
  connections:
  C/RConn1 -- RLC5/LConn1
  B/RConn1 -- RLC4/LConn1
  A/RConn1 -- RLC3/LConn1
  RLC3/RConn1 -- RLC2/LConn1
  RLC1/LConn1 -- RLC4/RConn1
  "RLC "/LConn1 -- RLC5/RConn1
  RLC2/RConn1 -- Ground2/LConn1 -- RLC1/RConn1 -- "RLC "/RConn1

== system Diesel_Genset_lib/4_MVA_Diesel_Generator/GenSet_4MVA_copy1mva/Simulated Generator Controller 3.5 MW ==
  Pref : Inport
  Qref : Inport  Port=2
  mode : Inport  Port=3
  set_vtref : Inport  Port=4
  set_wref : Inport  Port=5
  gen_m : Inport  Port=6
  Bus Selector1 : BusSelector  OutputSignals="Output active power   Peo (pu),Output reactive power  Qeo (pu)"
  Multiport Switch : MultiPortSwitch
  Mux1 : Mux  Inputs=2
  Mux2 : Mux  Inputs=2
  Mux3 : Mux  Inputs=2
  PQ control : Subsystem
  PV control : Subsystem
  "wref, Vref" : Outport
  wires:
  Bus Selector1/1 -> PQ control/2(P (pu)), PV control/2(P (pu))  "<Output active power   Peo (pu)>"
  gen_m/1 -> Bus Selector1/1
  PQ control/1(w_ref (pu)) -> Mux1/1
  PQ control/2(V_ref (pu)) -> Mux1/2
  PV control/1(w_ref (pu)) -> Mux2/1
  set_vtref/1 -> Mux2/2, Mux3/2
  Mux1/1 -> Multiport Switch/2
  Mux2/1 -> Multiport Switch/3
  Mux3/1 -> Multiport Switch/4
  Pref/1 -> PQ control/1(P_ref (pu)), PV control/1(P_ref (pu))
  Bus Selector1/2 -> PQ control/4(Q (pu))  "<Output reactive power  Qeo (pu)>"
  set_wref/1 -> Mux3/1
  Qref/1 -> PQ control/3(Q_ref (pu))
  mode/1 -> Multiport Switch/1
  Multiport Switch/1 -> "wref, Vref"/1

== system Diesel_Genset_lib/4_MVA_Diesel_Generator/GenSet_4MVA_copy1mva/StabilityL ==
  Constant Load : powerlib/Elements/Three-Phase Parallel RLC Load  LConnTagsString=A|B|C  Configuration=Y (grounded)  NominalVoltage=v  NominalFrequency=60  ActivePower=kVA*1E3*pf  InductivePower=kVA*1E3*sqrt(1-pf^2)  CapacitivePower=0  Measurements=None  LoadType=constant Z
  A : PMIOPort  Port=1  Side=Left
  B : PMIOPort  Port=2  Side=Left
  C : PMIOPort  Port=3  Side=Left
  connections:
  A/RConn1 -- Constant Load/LConn1
  B/RConn1 -- Constant Load/LConn2
  C/RConn1 -- Constant Load/LConn3

== system Diesel_Genset_lib/4_MVA_Diesel_Generator/Woodward Inputs/Speed_System ==
  In1 : Inport
  Clock1 : Clock
      settings: DisableCoverage=on
  Duty : Constant  DisableCoverage=on  Value=0.5
  Gain1 : Gain  Gain=5
  Gain3 : Gain  Gain=5
  Gain4 : Gain  Gain=1800
  Output : Trigonometry
  Product1 : Product  DisableCoverage=on  SaturateOnIntegerOverflow=on  InputSameDT=on  OutDataTypeStr=Inherit: Same as first input
  Product3 : Product  DisableCoverage=on  SaturateOnIntegerOverflow=on  InputSameDT=on  OutDataTypeStr=Inherit: Same as first input
  RTE Conversion : rteventslib/Signal Attributes/RTE Conversion  inputdatatype=RTE Boolean  outputdatatype=Double  compensation=Disabled  nbMaxEvents=10  sampleTime=Ts
  RTE SPWM : rteventslib/Sources/RTE SPWM  NumberPhases=1-ph  CenterAlignmentMode=On  MaxFreq=inf  MinFreq=0  EnablingPort=off  ComplementaryMode=off  SpaceVector=off  RiseTimeDelay=0  MaxEvents=10  SampleTime=Ts
  initialFreq : Constant  DisableCoverage=on  Value=2*pi
  Out1 : Outport
  wires:
  Product1/1 -> Output/1
  Clock1/1 -> Product1/1
  initialFreq/1 -> Product3/1
  Product3/1 -> Product1/2
  Gain4/1 -> Product3/2, RTE SPWM/1
  Output/1 -> Gain3/1
  In1/1 -> Gain4/1
  RTE SPWM/1 -> RTE Conversion/1
  Duty/1 -> RTE SPWM/2
  RTE Conversion/1 -> Gain1/1
  Gain1/1 -> Out1/1

== system Diesel_Genset_lib/4_MVA_Diesel_Generator/Woodward Inputs/Speed_System1 ==
  In1 : Inport
  Clock1 : Clock
      settings: DisableCoverage=on
  Duty : Constant  DisableCoverage=on  Value=0.5
  Gain1 : Gain  Gain=5
  Gain3 : Gain  Gain=5
  Gain4 : Gain  Gain=1800
  Output : Trigonometry
  Product1 : Product  DisableCoverage=on  SaturateOnIntegerOverflow=on  InputSameDT=on  OutDataTypeStr=Inherit: Same as first input
  Product3 : Product  DisableCoverage=on  SaturateOnIntegerOverflow=on  InputSameDT=on  OutDataTypeStr=Inherit: Same as first input
  RTE Conversion : rteventslib/Signal Attributes/RTE Conversion  inputdatatype=RTE Boolean  outputdatatype=Double  compensation=Disabled  nbMaxEvents=10  sampleTime=Ts
  RTE SPWM : rteventslib/Sources/RTE SPWM  NumberPhases=1-ph  CenterAlignmentMode=On  MaxFreq=inf  MinFreq=0  EnablingPort=off  ComplementaryMode=off  SpaceVector=off  RiseTimeDelay=0  MaxEvents=10  SampleTime=Ts
  initialFreq : Constant  DisableCoverage=on  Value=2*pi
  Out1 : Outport
  wires:
  Product1/1 -> Output/1
  Clock1/1 -> Product1/1
  initialFreq/1 -> Product3/1
  Product3/1 -> Product1/2
  Gain4/1 -> Product3/2, RTE SPWM/1
  Output/1 -> Gain3/1
  In1/1 -> Gain4/1
  RTE SPWM/1 -> RTE Conversion/1
  Duty/1 -> RTE SPWM/2
  RTE Conversion/1 -> Gain1/1
  Gain1/1 -> Out1/1

== system Diesel_Genset_lib/4_MVA_Diesel_Generator/Woodward Outputs/DIO - Gr3 ==
  Dout : Inport
  Bus Creator : BusCreator  Inputs=1
  Bus Selector1 : BusSelector  OutputSignals=DI_CH08-15  OutputAsBus=on
  Conditioning1 : Subsystem
  DigitalIn1 : rtio_opalrt_common/DigitalIn  CtrlName='OpCtrl'  portNb=6  FcnNos=Slot 3 Module A Subsection 2  size=1  maxcount=8  count=8  sampleTime=0  numchan=8
      settings: AttributesFormatString=%<CtrlName>
  DigitalOut1 : rtio_opalrt_common/DigitalOut  CtrlName='OpCtrl'  portNb=6  FcnNos=Slot 3 Module B Subsection 2  size=1  maxcount=8  count=8  numchan=8
      settings: AttributesFormatString=%<CtrlName>
  Terminator1 : Terminator
  Terminator6 : Terminator
  DIn : Outport
  wires:
  Conditioning1/1(Out1) -> Bus Creator/1
  Bus Creator/1 -> DIn/1
  DigitalIn1/1 -> Conditioning1/1(In1)  "DI_CH08-15"
  DigitalIn1/2 -> Terminator6/1
  Bus Selector1/1 -> DigitalOut1/1
  Dout/1 -> Bus Selector1/1
  DigitalOut1/1 -> Terminator1/1

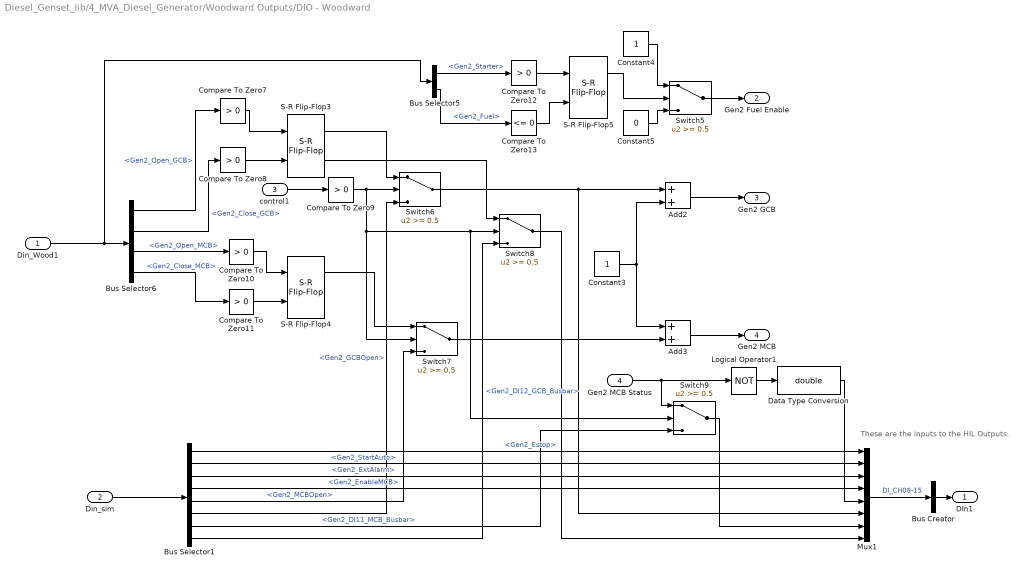
== system Diesel_Genset_lib/4_MVA_Diesel_Generator/Woodward Outputs/DIO - Woodward ==
  note: These are the inputs to
      | the HIL Outputs.
  Din_Wood1 : Inport
  Din_sim : Inport  Port=2
  control1 : Inport  Port=3
  Gen2 MCB Status : Inport  Port=4
  Add2 : Sum
  Add3 : Sum
  Bus Creator : BusCreator  Inputs=1
  Bus Selector1 : BusSelector  OutputSignals=16 DOUT GR3.08-11.Gen2_Estop,16 DOUT GR3.08-11.Gen2_StartAuto,16 DOUT GR3.08-11.Gen2_ExtAlarm,16 DOUT GR3.08-11.Gen2_EnableMCB,16 DOUT GR3.12-15.Gen2_MCBOpen,16 DOUT GR3.12-15.Gen2_GCBOpen,16 DOUT GR3.12-15.Gen2_DI11_MCB_Busbar,16 DOUT GR3.12-15.Gen2_DI12_GCB_Busbar
  Bus Selector5 : BusSelector  OutputSignals=DI_CH08-15.Gen2_Starter,DI_CH08-15.Gen2_Fuel
  Bus Selector6 : BusSelector  OutputSignals=DI_CH08-15.Gen2_Open_GCB,DI_CH08-15.Gen2_Close_GCB,DI_CH08-15.Gen2_Open_MCB,DI_CH08-15.Gen2_Close_MCB
  Compare To Zero{7..12} (6 alike) : simulink/Logic and Bit Operations/Compare To Zero  relop=>  OutDataTypeStr=boolean
  Compare To Zero13 : simulink/Logic and Bit Operations/Compare To Zero  relop=<=  OutDataTypeStr=boolean
  Constant3 : Constant
  Constant4 : Constant
  Constant5 : Constant  Value=0
  Data Type Conversion : DataTypeConversion  OutDataTypeStr=double
  Logical Operator1 : Logic  Operator=NOT  AllPortsSameDT=off  OutDataTypeStr=boolean
  Mux1 : Mux  Inputs=8
  S-R Flip-Flop3 : simulink_extras/Flip Flops/S-R Flip-Flop  initial_condition=1
  S-R Flip-Flop4 : simulink_extras/Flip Flops/S-R Flip-Flop  initial_condition=1
  S-R Flip-Flop5 : simulink_extras/Flip Flops/S-R Flip-Flop  initial_condition=0
  Switch5 : Switch  Threshold=0.5
  Switch{6..9} (4 alike) : Switch  Threshold=0.5  OutDataTypeStr=double
      Switch8 settings: LockScale=on
  DIn1 : Outport
  Gen2 Fuel Enable : Outport  Port=2
  Gen2 GCB : Outport  Port=3
  Gen2 MCB : Outport  Port=4
  wires:
  Data Type Conversion/1 -> Mux1/5
  Logical Operator1/1 -> Data Type Conversion/1
  Gen2 MCB Status/1 -> Switch9/1, Logical Operator1/1
  Switch8/1 -> Mux1/8
  Bus Selector1/8 -> Switch8/3  "<Gen2_DI12_GCB_Busbar>"
  Switch9/1 -> Mux1/7
  Bus Selector1/7 -> Switch9/3  "<Gen2_DI11_MCB_Busbar>"
  Din_sim/1 -> Bus Selector1/1
  Bus Selector1/6 -> Switch6/3  "<Gen2_GCBOpen>"
  Bus Selector1/5 -> Switch7/3  "<Gen2_MCBOpen>"
  Bus Selector1/4 -> Mux1/4  "<Gen2_EnableMCB>"
  Bus Selector1/3 -> Mux1/3  "<Gen2_ExtAlarm>"
  Bus Selector1/2 -> Mux1/2  "<Gen2_StartAuto>"
  Bus Selector1/1 -> Mux1/1  "<Gen2_Estop>"
  Switch5/1 -> Gen2 Fuel Enable/1
  Compare To Zero13/1 -> S-R Flip-Flop5/2
  Constant4/1 -> Switch5/1
  Constant5/1 -> Switch5/3
  Compare To Zero12/1 -> S-R Flip-Flop5/1
  S-R Flip-Flop5/1 -> Switch5/2
  Bus Selector5/2 -> Compare To Zero13/1  "<Gen2_Fuel>"
  Bus Selector5/1 -> Compare To Zero12/1  "<Gen2_Starter>"
  Constant3/1 -> Add3/1, Add2/2
  Add3/1 -> Gen2 MCB/1
  Add2/1 -> Gen2 GCB/1
  S-R Flip-Flop3/2 -> Switch8/1
  Switch7/1 -> Add3/2
  Compare To Zero9/1 -> Switch9/2, Switch8/2, Switch7/2, Switch6/2
  Bus Selector6/2 -> Compare To Zero8/1  "<Gen2_Close_GCB>"
  S-R Flip-Flop4/1 -> Switch7/1
  Compare To Zero10/1 -> S-R Flip-Flop4/1
  Bus Selector6/3 -> Compare To Zero10/1  "<Gen2_Open_MCB>"
  Compare To Zero11/1 -> S-R Flip-Flop4/2
  Bus Selector6/4 -> Compare To Zero11/1  "<Gen2_Close_MCB>"
  Compare To Zero8/1 -> S-R Flip-Flop3/2
  Compare To Zero7/1 -> S-R Flip-Flop3/1
  Bus Selector6/1 -> Compare To Zero7/1  "<Gen2_Open_GCB>"
  Switch6/1 -> Mux1/6, Add2/1
  S-R Flip-Flop3/1 -> Switch6/1
  control1/1 -> Compare To Zero9/1
  Mux1/1 -> Bus Creator/1  "DI_CH08-15"
  Bus Creator/1 -> DIn1/1
  Din_Wood1/1 -> Bus Selector6/1, Bus Selector5/1

== system Diesel_Genset_lib/4_MVA_Diesel_Generator/Woodward Outputs/DOUT type config ==
  note: The Constants are used to select Digital Output type:
      | - 0: Time-Stamped Digital Output
      | - 1: Pulse-Width Modulated DIgital Output
  DataIn Send : rtio_opalrt_common/DataIn Send  CtrlName='OpCtrl'  FcnNos=11  width=1  portType=double  checkVersion=off  expectedId=0  expectedVersion=0  opComp=>=
      settings: AttributesFormatString=%<CtrlName>
  DataIn Send1 : rtio_opalrt_common/DataIn Send  CtrlName='OpCtrl'  FcnNos=12  width=1  portType=double  checkVersion=off  expectedId=0  expectedVersion=0  opComp=>=
      settings: AttributesFormatString=%<CtrlName>
  Subsection 3 DOUT type : Constant
  Subsection 4 DOUT type : Constant
  Terminator1 : Terminator
  Terminator2 : Terminator
  wires:
  DataIn Send/1 -> Terminator2/1
  DataIn Send1/1 -> Terminator1/1
  Subsection 4 DOUT type/1 -> DataIn Send1/1
  Subsection 3 DOUT type/1 -> DataIn Send/1

== system Diesel_Genset_lib/4_MVA_Diesel_Generator/Woodward Outputs/PWM IO - Gr3 ==
  PWMOut : Inport
  Bus Creator : BusCreator  Inputs=2
  Bus Creator1 : BusCreator  Inputs=2
  Bus Creator2 : BusCreator  Inputs=2
  Bus Selector : BusSelector  OutputSignals=FreqPWMOut16-23,DutyPWMOut16-23
  Bus Selector1 : BusSelector  OutputSignals=FreqPWMOut24-31,DutyPWMOut24-31
  Bus Selector2 : BusSelector  OutputSignals=16 PWMOUT GR3.Ch16-23,16 PWMOUT GR3.Ch24-31
  PWM In : rtio_opalrt_common/PWM In  CtrlName='OpCtrl'  portNb=9  FcnNos=Slot 3 Module A Subsection 3  maxCount=8  Count=8  sampleTime=0  numchan=8
      settings: AttributesFormatString=%<CtrlName>
  PWM In1 : rtio_opalrt_common/PWM In  CtrlName='OpCtrl'  portNb=10  FcnNos=Slot 3 Module A Subsection 4  maxCount=8  Count=8  sampleTime=0  numchan=8
      settings: AttributesFormatString=%<CtrlName>
  PWM Out : rtio_opalrt_common/PWM Out  CtrlName='OpCtrl'  portNb=9  FcnNos=Slot 3 Module B Subsection 3  size=64  maxcount=8  count=8  polarity=Active High  symMode=Symmetric  complementary=off  deadTime=0  numchan=8  loadnb=1  initphase=[0 0 0 0 0 0 0 0]
      settings: AttributesFormatString=%<CtrlName>
  PWM Out1 : rtio_opalrt_common/PWM Out  CtrlName='OpCtrl'  portNb=10  FcnNos=Slot 3 Module B Subsection 4  size=64  maxcount=8  count=8  polarity=Active High  symMode=Symmetric  complementary=off  deadTime=0  numchan=8  loadnb=2  initphase=[0 0 0 0 0 0 0 0]
      settings: AttributesFormatString=%<CtrlName>
  Terminator{,1,4..5} (4 alike) : Terminator
  PWMIn : Outport
  wires:
  Bus Selector2/2 -> Bus Selector1/1  "<Ch24-31>"
  PWM In1/2 -> Bus Creator2/2  "Duty"
  PWM In1/1 -> Bus Creator2/1  "Freq"
  PWM In/2 -> Bus Creator1/2  "Duty"
  PWM In/1 -> Bus Creator1/1  "Freq"
  PWM In/3 -> Terminator4/1
  PWM In1/3 -> Terminator5/1
  Bus Creator2/1 -> Bus Creator/2  "PWMI_CH24-31"
  Bus Creator1/1 -> Bus Creator/1  "PWMI_CH16-23"
  Bus Creator/1 -> PWMIn/1
  Bus Selector2/1 -> Bus Selector/1  "<Ch16-23>"
  PWMOut/1 -> Bus Selector2/1
  PWM Out1/1 -> Terminator1/1
  Bus Selector1/2 -> PWM Out1/2  "<DutyPWMOut24-31>"
  Bus Selector1/1 -> PWM Out1/1  "<FreqPWMOut24-31>"
  PWM Out/1 -> Terminator/1
  Bus Selector/2 -> PWM Out/2  "<DutyPWMOut16-23>"
  Bus Selector/1 -> PWM Out/1  "<FreqPWMOut16-23>"
